simulink model "parallel_lht"  (R2019b)
settings: Solver=FixedStepDiscrete  StartTime=0.0  StopTime=inf  RelTol=1e-3
undefined symbols (not defined in the file or in its folder): bt, height, nTheta, width
libraries: hdlsllib x21, simulink x18, dspsrcs4 x1
(part 2 of 2)

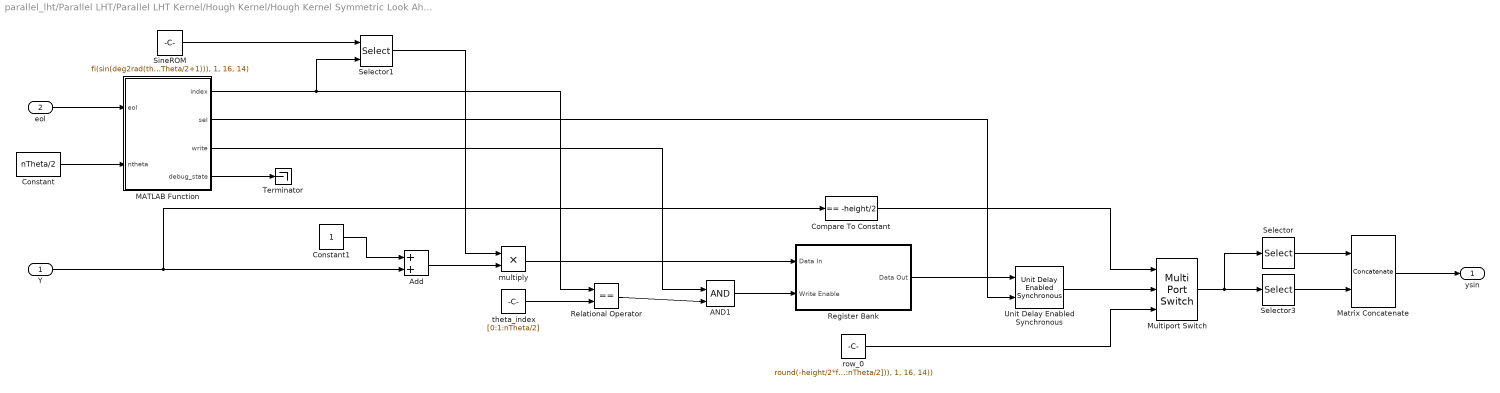
== system parallel_lht/Parallel LHT/Parallel LHT Kernel/Hough Kernel/Hough Kernel Symmetric Look Ahead/Look Ahead Hough ==
  Y : Inport
  eol : Inport  Port=2
  AND1 : Logic  IconShape=distinctive  AllPortsSameDT=off  OutDataTypeStr=boolean
  Add : Sum  OutDataTypeStr=fixdt(1,ceil(log2(height)),0)
  Compare To Constant : simulink/Logic and Bit Operations/Compare To Constant  relop===  const=-height/2  OutDataTypeStr=boolean
  Constant : Constant  Value=nTheta/2  OutDataTypeStr=fixdt(0, ceil(log2(nTheta+1)), 0)  SampleTime=-1
  Constant1 : Constant  OutDataTypeStr=fixdt(1, ceil(log2(height)), 0);  SampleTime=-1
  MATLAB Function : MATLAB Function  TreatAsAtomicUnit=on
  Matrix Concatenate : Concatenate  Mode=Multidimensional array  ConcatenateDimension=2
  Multiport Switch : MultiPortSwitch  DataPortOrder=Zero-based contiguous  Inputs=2  zeroidx=on
  Register Bank : Subsystem  TreatAsAtomicUnit=on
  Relational Operator : RelationalOperator  Operator===  OutDataTypeStr=boolean  RndMeth=Simplest
  Selector : Selector  NumberOfDimensions=2  IndexMode=Zero-based  InputPortWidth=3  IndexOptions=Index vector (dialog),Index vector (dialog)  Indices=0,[0:1:nTheta/2-1]  OutputSizes=1,1
  Selector1 : Selector  NumberOfDimensions=2  IndexMode=Zero-based  InputPortWidth=3  IndexOptions=Index vector (dialog),Index vector (port)  Indices=0,1  OutputSizes=1,1
  Selector3 : Selector  NumberOfDimensions=2  IndexMode=Zero-based  InputPortWidth=3  IndexOptions=Index vector (dialog),Index vector (dialog)  Indices=0,nTheta/2  OutputSizes=1,1
  SineROM : Constant  Value=fi(sin(deg2rad(theta(1:1:nTheta/2+1))), 1, 16, 14)  VectorParams1D=off  OutDataTypeStr=fixdt(1,16,14)  SampleTime=-1
  Terminator : Terminator
  Unit Delay Enabled Synchronous : hdlsllib/Discrete/Unit Delay Enabled Synchronous  InitialCondition=0.0  SampleTime=-1
      settings: SourceProductName=Simulink  SourceProductBaseCode=SL
  multiply : Product  OutDataTypeStr=fixdt(1, ceil(log2(height)), 0);  RndMeth=Round
  row_0 : Constant  Value=round(-height/2*fi(sin(deg2rad([0:1:nTheta/2])), 1, 16, 14))  VectorParams1D=off  OutDataTypeStr=fixdt(1,ceil(log2(height)),0)  SampleTime=-1
  theta_index : Constant  Value=[0:1:nTheta/2]  VectorParams1D=off  OutDataTypeStr=fixdt(0,ceil(log2(max(theta)+1)),0)  SampleTime=-1
  ysin : Outport  VectorParamsAs1DForOutWhenUnconnected=off
  wires:
  Multiport Switch/1 -> Selector3/1, Selector/1
  Unit Delay Enabled Synchronous/1 -> Multiport Switch/2
  Register Bank/1(Data Out) -> Unit Delay Enabled Synchronous/1
  Compare To Constant/1 -> Multiport Switch/1
  MATLAB Function/2(sel) -> Unit Delay Enabled Synchronous/2
  SineROM/1 -> Selector1/1
  Matrix Concatenate/1 -> ysin/1
  Selector3/1 -> Matrix Concatenate/2
  Selector/1 -> Matrix Concatenate/1
  MATLAB Function/4(debug_state) -> Terminator/1
  AND1/1 -> Register Bank/2(Write Enable)
  Relational Operator/1 -> AND1/2
  theta_index/1 -> Relational Operator/2
  multiply/1 -> Register Bank/1(Data In)
  Selector1/1 -> multiply/1
  MATLAB Function/1(index) -> Relational Operator/1, Selector1/2
  eol/1 -> MATLAB Function/1(eol)
  Constant/1 -> MATLAB Function/2(ntheta)
  MATLAB Function/3(write) -> AND1/1
  Constant1/1 -> Add/1
  Y/1 -> Compare To Constant/1, Add/2
  Add/1 -> multiply/2
  row_0/1 -> Multiport Switch/3

== system parallel_lht/Parallel LHT/Parallel LHT Accumulator/Accumulator with Switches/Accumulator/Block RAM/Simple Dual Port RAM ==
  wr_data : Inport
  wr_addr : Inport  Port=2
  wr_en : Inport  Port=3
  rd_addr : Inport  Port=4
  Simple Dual Port RAM : hdlsllib/HDL RAMs/Simple Dual Port RAM  ram_size=ceil(log2(maxRho*2))
      settings: SourceProductName=Simulink  SourceProductBaseCode=SL
  rd_data : Outport
  wires:
  wr_data/1 -> Simple Dual Port RAM/1
  wr_addr/1 -> Simple Dual Port RAM/2
  wr_en/1 -> Simple Dual Port RAM/3
  rd_addr/1 -> Simple Dual Port RAM/4
  Simple Dual Port RAM/1 -> rd_data/1

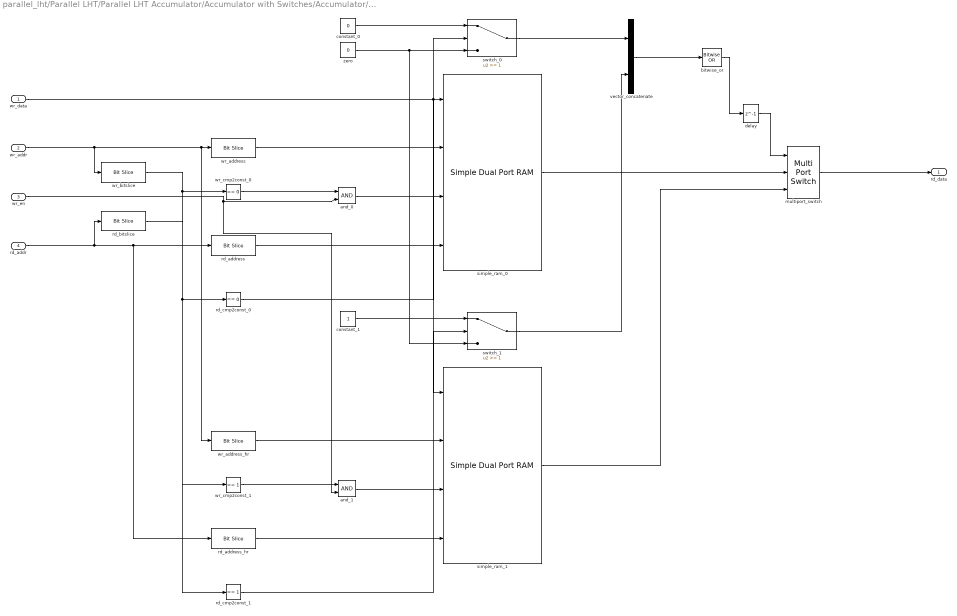
== system parallel_lht/Parallel LHT/Parallel LHT Accumulator/Accumulator with Switches/Accumulator/Block RAM/Simple Dual Port RAM Generator ==
  wr_data : Inport
  wr_addr : Inport  Port=2
  wr_en : Inport  Port=3
  rd_addr : Inport  Port=4
  and_0 : Logic  AllPortsSameDT=off  OutDataTypeStr=boolean
  and_1 : Logic  AllPortsSameDT=off  OutDataTypeStr=boolean
  bitwise_or : simulink/Logic and Bit Operations/Bitwise Operator  logicop=OR  UseBitMask=off  BitMask=bin2dec('11011001')  BitMaskRealWorld=Stored Integer
  constant_0 : Constant  Value=0  OutDataTypeStr=fixdt(0, 2, 0)  SampleTime=-1
  constant_1 : Constant  OutDataTypeStr=fixdt(0, 2, 0)  SampleTime=-1
  delay : Delay  DelayLength=1
  multiport_switch : MultiPortSwitch  DataPortOrder=Zero-based contiguous  Inputs=2  zeroidx=on
  rd_address : hdlsllib/Logic and Bit Operations/Bit Slice  lidx=10  ridx=0
      settings: SourceProductName=Simulink  SourceProductBaseCode=SL
  rd_address_hr : hdlsllib/Logic and Bit Operations/Bit Slice  lidx=9  ridx=0
      settings: SourceProductName=Simulink  SourceProductBaseCode=SL
  rd_bitslice : hdlsllib/Logic and Bit Operations/Bit Slice  lidx=11  ridx=11
      settings: SourceProductName=Simulink  SourceProductBaseCode=SL
  rd_cmp2const_0 : simulink/Logic and Bit Operations/Compare To Constant  relop===  const=0  OutDataTypeStr=boolean
  rd_cmp2const_1 : simulink/Logic and Bit Operations/Compare To Constant  relop===  const=1  OutDataTypeStr=boolean
  simple_ram_0 : hdlsllib/HDL RAMs/Simple Dual Port RAM  ram_size=11
      settings: SourceProductName=Simulink  SourceProductBaseCode=SL
  simple_ram_1 : hdlsllib/HDL RAMs/Simple Dual Port RAM  ram_size=10
      settings: SourceProductName=Simulink  SourceProductBaseCode=SL
  switch_0 : Switch  Threshold=1
  switch_1 : Switch  Threshold=1
  vector_concatenate : Concatenate
  wr_address : hdlsllib/Logic and Bit Operations/Bit Slice  lidx=10  ridx=0
      settings: SourceProductName=Simulink  SourceProductBaseCode=SL
  wr_address_hr : hdlsllib/Logic and Bit Operations/Bit Slice  lidx=9  ridx=0
      settings: SourceProductName=Simulink  SourceProductBaseCode=SL
  wr_bitslice : hdlsllib/Logic and Bit Operations/Bit Slice  lidx=11  ridx=11
      settings: SourceProductName=Simulink  SourceProductBaseCode=SL
  wr_cmp2const_0 : simulink/Logic and Bit Operations/Compare To Constant  relop===  const=0  OutDataTypeStr=boolean
  wr_cmp2const_1 : simulink/Logic and Bit Operations/Compare To Constant  relop===  const=1  OutDataTypeStr=boolean
  zero : Constant  Value=0  OutDataTypeStr=fixdt(0, 2, 0)  SampleTime=-1
  rd_data : Outport
  wires:
  wr_data/1 -> simple_ram_0/1, simple_ram_1/1
  wr_address/1 -> simple_ram_0/2
  rd_address/1 -> simple_ram_0/4
  constant_0/1 -> switch_0/1
  zero/1 -> switch_0/3, switch_1/3
  switch_0/1 -> vector_concatenate/1
  simple_ram_0/1 -> multiport_switch/2
  wr_bitslice/1 -> wr_cmp2const_0/1, wr_cmp2const_1/1
  rd_bitslice/1 -> rd_cmp2const_0/1, rd_cmp2const_1/1
  wr_en/1 -> and_0/2, and_1/2
  and_0/1 -> simple_ram_0/3
  wr_cmp2const_0/1 -> and_0/1
  rd_cmp2const_0/1 -> switch_0/2
  constant_1/1 -> switch_1/1
  switch_1/1 -> vector_concatenate/2
  simple_ram_1/1 -> multiport_switch/3
  and_1/1 -> simple_ram_1/3
  wr_cmp2const_1/1 -> and_1/1
  rd_cmp2const_1/1 -> switch_1/2
  rd_addr/1 -> rd_address/1, rd_address_hr/1, rd_bitslice/1
  wr_addr/1 -> wr_address/1, wr_address_hr/1, wr_bitslice/1
  vector_concatenate/1 -> bitwise_or/1
  bitwise_or/1 -> delay/1
  delay/1 -> multiport_switch/1
  multiport_switch/1 -> rd_data/1
  wr_address_hr/1 -> simple_ram_1/2
  rd_address_hr/1 -> simple_ram_1/4

== system parallel_lht/Parallel LHT/Parallel LHT Kernel/Hough Kernel/Hough Kernel Symmetric Look Ahead/Look Ahead Hough/Register Bank ==
  Data In : Inport
  Write Enable : Inport  Port=2  Partition=on  PartitionDimension=2  PartitionWidth=1  PartitionOffset=0
  For Each : ForEach  DisableCoverage=on
  Unit Delay Enabled Synchronous : hdlsllib/Discrete/Unit Delay Enabled Synchronous  InitialCondition=0.0  SampleTime=-1
      settings: SourceProductName=Simulink  SourceProductBaseCode=SL
  Data Out : Outport  ConcatenationDimension=2
  wires:
  Data In/1 -> Unit Delay Enabled Synchronous/1
  Unit Delay Enabled Synchronous/1 -> Data Out/1
  Write Enable/1 -> Unit Delay Enabled Synchronous/2

== matlab function parallel_lht/Parallel LHT/Parallel LHT Accumulator/Accumulator Controller ==
  data: sof input; mode output; eof input; read output; clear output; index output; ntheta input; nrho input; valid output
function [mode, read, clear, index, valid] = fcn(sof, eof, ntheta, nrho)

IDLE = fi(0, 0, 2, 0);
VOTE = fi(1, 0, 2, 0);
READ = fi(2, 0, 2, 0);
CLEAR = fi(3, 0, 2, 0);

persistent current_state;
persistent rho_counter;
persistent theta_counter;

if isempty(current_state)
    current_state = IDLE;
end

if isempty(rho_counter)
    rho_counter = fi(0, 0, 16, 0);
end

if isempty(theta_counter)
    theta_counter = fi(0, 0, 16, 0);
end

switch current_state
    case IDLE
        rho_counter = fi(0, 0, 16, 0);
        theta_counter = fi(0, 0, 16, 0);
        
        clear = false;
        read = rho_counter;
        index = theta_counter;
        valid = false;
        
        if sof
            mode = true;
            current_state = VOTE;
        else
            mode = false;
            current_state = IDLE;
        end
        
    case VOTE
        rho_counter = fi(0, 0, 16, 0);
        theta_counter = fi(0, 0, 16, 0);
        
        mode = true;
        clear = false;
        valid = false;
        
        read = rho_counter;
        index = theta_counter;
        
        if eof
            current_state = READ;
        else
            current_state = VOTE;
        end
        
    case READ
        mode = false;
        clear = false;
        read = rho_counter;
        index = theta_counter;
        valid = true;
        
        if theta_counter >= nrho && rho_counter >= ntheta
            rho_counter = fi(0, 0, 16, 0);
            theta_counter = fi(0, 0, 16, 0);
            current_state = CLEAR;
        elseif rho_counter >= nrho
            theta_counter = fi(theta_counter + 1, 0, 16, 0);
            rho_counter = fi(0, 0, 16, 0);
            current_state = READ;
        else
            rho_counter = fi(rho_counter + 1, 0, 16, 0);
            current_state = READ;
        end
        
    case CLEAR
        mode = false;
        clear = true;
        valid = false;
        
        read = rho_counter;
        index = theta_counter;
        
        if rho_counter >= nrho
            rho_counter = fi(0, 0, 16, 0);
            theta_counter = fi(0, 0, 16, 0);
            current_state = IDLE;
        else
            rho_counter = fi(rho_counter + 1, 0, 16, 0);
            theta_counter = fi(0, 0, 16, 0);
            current_state = CLEAR;
        end
        
    otherwise
        rho_counter = fi(0, 0, 16, 0);
        theta_counter = fi(0, 0, 16, 0);
        
        mode = false;
        clear = false;
        valid = false;
        
        read = rho_counter;
        index = theta_counter;
        
        current_state = IDLE;
        
end

== matlab function parallel_lht/Parallel LHT/Parallel LHT Kernel/Hough Kernel/Hough Kernel Symmetric Look Ahead/Look Ahead Hough/MATLAB Function ==
  data: index output; eol input; sel output; write output; ntheta input; debug_state output
function [index, sel, write, debug_state] = fcn(eol, ntheta)

BANK = fi(1, 0, 3, 0);
WAIT = fi(2, 0, 3, 0);

persistent state;

persistent thetacounter;

if isempty(state)
    state = BANK;
end

if isempty(thetacounter)
    thetacounter = fi(0, 0, 16, 0);
end

switch state
    case BANK
        sel = false;
        write = true;
        index = thetacounter;
        debug_state = state;
        
        if thetacounter == ntheta
            thetacounter = fi(0, 0, 16, 0);
            state = WAIT;
        else
            thetacounter = fi(thetacounter + 1, 0, 16, 0);
            state = BANK;
        end
        
    case WAIT
        write = false;
        index = thetacounter;
        debug_state = state;
        
        thetacounter = fi(0, 0, 16, 0);
        
        if eol
            sel = true;
            state = BANK;
        else
            sel = false;
            state = WAIT;
        end
        
    otherwise
        thetacounter = fi(0, 0, 16, 0);
        sel = false;
        write = false;
        index = thetacounter;
        debug_state = state;
        
        state = WAIT;
        
end
